simulink model "Crane3D"  (R2024b)
settings: Solver=ode4  StartTime=0.0  StopTime=Tsim  FixedStep=0.01  RelTol=1e-3  AbsTol=1e-6
values from neighbouring files (symbols this model uses):
  den_X = pCartd_X.den{1}    [script_3DCrane.m]
  den_Y = pCartd_Y.den{1}    [script_3DCrane.m]
  den_Z = pCartd_Z.den{1}    [script_3DCrane.m]
  num_X = pCartd_X.num{1}    [script_3DCrane.m]
  num_Y = pCartd_Y.num{1}    [script_3DCrane.m]
  num_Z = pCartd_Z.num{1}    [script_3DCrane.m]
  Ts = 0.01    [script_3DCrane.m]
libraries: simulink x1
settings Model: ExtModeTrigDuration=10000  Creator=jims  LastModifiedBy=David
settings SolverCC: AutoScaleAbsTol=off  AlgebraicLoopSolver=TrustRegion
settings DataIOCC: ExternalInput=[]  InitialState=[]  MaxDataPoints=5000  SaveFormat=Array  SaveOutput=off  SaveTime=off  ReturnWorkspaceOutputs=off
settings OptimizationCC: BooleanDataType=off  OptimizeBlockIOStorage=off  BufferReuse=off  GlobalBufferReuse=off  ExpressionFolding=off  ExpressionDepthLimit=2147483647  LocalBlockOutputs=off  InitFltsAndDblsToZero=on  LifeSpan=inf  OptimizeDataStoreBuffers=off  BusAssignmentInplaceUpdate=off
settings DebuggingCC: SaveWithParameterizedLinksMsg=none  UnderspecifiedInitializationDetection=Classic  MergeDetectMultiDrivingBlocksExec=none  SignalResolutionControl=TryResolveAllWithWarning  MultiTaskDSMMsg=warning  MultiTaskCondExecSysMsg=none  IntegerOverflowMsg=none  FcnCallInpInsideContextMsg=warning  UnconnectedInputMsg=warning  UnconnectedOutputMsg=warning  UnconnectedLineMsg=warning  StateNameClashWarn=warning  SFUnexpectedBacktrackingDiag=warning  SFNoUnconditionalDefaultTransitionDiag=warning  SFExecutionAtInitializationDiag=none  IntegerSaturationMsg=none  ArithmeticOperatorsInVariantConditions=warning
settings HardwareCC: ProdBitPerPointer=32  ProdBitPerSizeT=32  ProdBitPerPtrDiffT=32  ProdLargestAtomicFloat=None  ProdIntDivRoundTo=Undefined  ProdEndianess=Unspecified  ProdWordSize=32  ProdHWDeviceType=32-bit Generic
settings ModelReferenceCC: EnableRefExpFcnMdlSchedulingChecks=on  PropagateSignalLabelsOutOfModel=off
settings SFSimCC: SimUseLocalCustomCode=off  CustomCodeUndefinedFunction=UseInterfaceOnly
settings RTWCC: RTWUseLocalCustomCode=off  GPUComputeCapability=3.5
settings CodeAppCC: StateflowObjectComments=on
settings GRTTargetCC: TargetFcnLib=ansi_tfl_tmw.mat  TargetLangStandard=C89/C90 (ANSI)  CombineOutputUpdateFcns=off  GRTInterface=on
settings ConfigComp: CovMetricSettings=dw  CovSaveCumulativeToWorkspaceVar=on  CovSaveSingleToWorkspaceVar=on  CovExternalEMLEnable=off

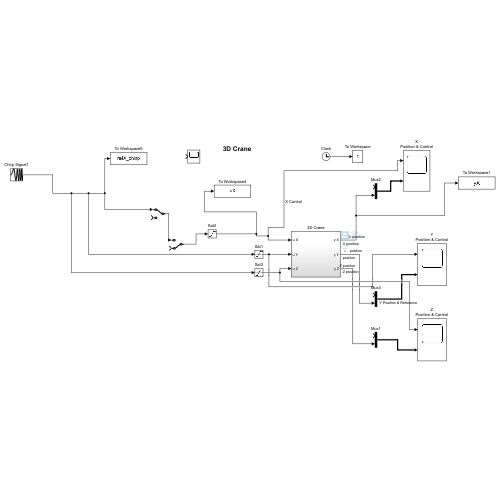
[thumbnail: Simulink's stored preview of the top-level diagram]
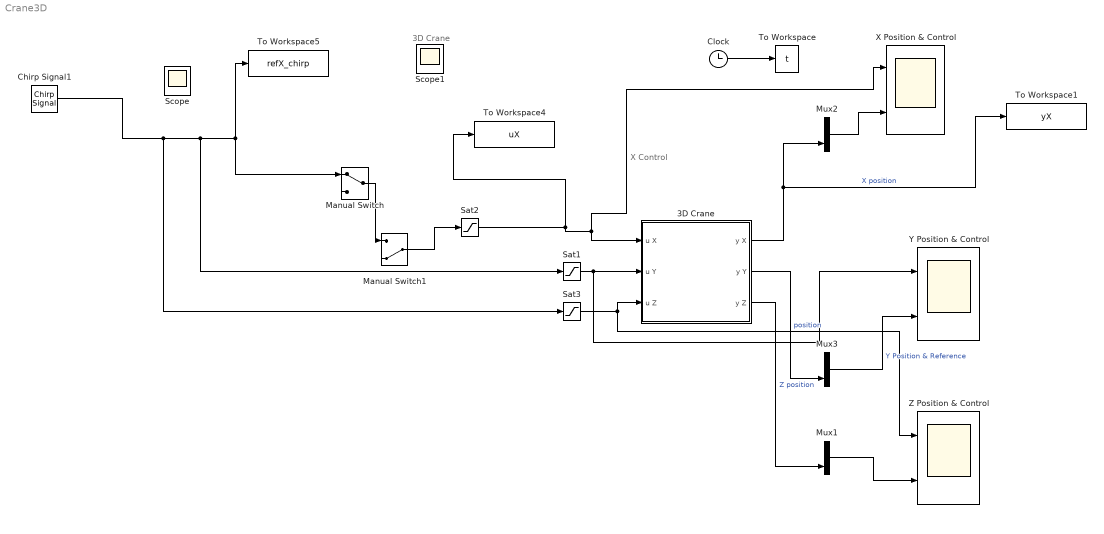
== system Crane3D ==
  note: 3D Crane
  note: X Control
  3D Crane : Subsystem
  Chirp Signal1 : simulink/Sources/Chirp Signal  f1=0.1  T=100  f2=1
  Clock : Clock
  Manual Switch : ManualSwitch
  Manual Switch1 : ManualSwitch  CurrentSetting=0
  Mux1 : Mux  Inputs=2
  Mux2 : Mux  Inputs=2
  Mux3 : Mux  Inputs=2
  Sat1 : Saturate  UpperLimit=1  LowerLimit=-1  SampleTime=Ts
  Sat2 : Saturate  UpperLimit=1  LowerLimit=-1  SampleTime=Ts
  Sat3 : Saturate  UpperLimit=1  LowerLimit=-1  SampleTime=Ts
  Scope1 : Scope
  To Workspace : ToWorkspace  VariableName=t  SampleTime=Ts
  To Workspace1 : ToWorkspace  VariableName=yX  SampleTime=Ts
      settings: Save2DSignal=2-D array (concatenate along first dimension)
  To Workspace4 : ToWorkspace  VariableName=uX  SampleTime=Ts
      settings: Save2DSignal=2-D array (concatenate along first dimension)
  To Workspace5 : ToWorkspace  VariableName=refX_chirp  SampleTime=Ts
      settings: Save2DSignal=2-D array (concatenate along first dimension)
  X Position & Control : Scope  NumInputPorts=2
  Y Position & Control : Scope  NumInputPorts=2
  Z Position & Control : Scope  NumInputPorts=2
  Scope : Scope
  wires:
  Mux2/1 -> X Position & Control/2
  Mux3/1 -> Y Position & Control/2  "Y Position & Reference"
  Clock/1 -> To Workspace/1
  Sat2/1 -> 3D Crane/1(u X), X Position & Control/1, To Workspace4/1
  Sat1/1 -> Y Position & Control/1, 3D Crane/2(u Y)
  Sat3/1 -> 3D Crane/3(u Z), Z Position & Control/1
  Mux1/1 -> Z Position & Control/2
  3D Crane/1(y X) -> To Workspace1/1, Mux2/2  "X position"
  3D Crane/2(y Y) -> Mux3/2  "position"
  3D Crane/3(y Z) -> Mux1/2  "Z position"
  Chirp Signal1/1 -> Sat3/1, Sat1/1, To Workspace5/1, Manual Switch/1
  Manual Switch/1 -> Manual Switch1/1
  Manual Switch1/1 -> Sat2/1

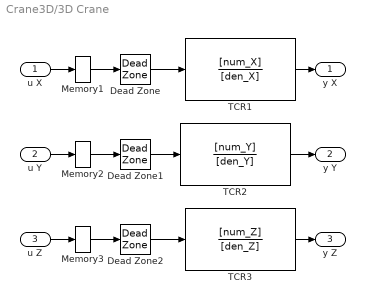
== system Crane3D/3D Crane ==
  u X : Inport
  u Y : Inport  Port=2
  u Z : Inport  Port=3
  Dead Zone : DeadZone  LowerValue=DZmin_X  UpperValue=DZmax_X
  Dead Zone1 : DeadZone  LowerValue=DZmin_Y  UpperValue=DZmax_Y
  Dead Zone2 : DeadZone  LowerValue=DZmin_Z  UpperValue=DZmax_Z
  Memory1 : Memory
  Memory2 : Memory
  Memory3 : Memory
  TCR1 : DiscreteTransferFcn  Numerator=[num_X]  Denominator=[den_X]  SampleTime=Ts
  TCR2 : DiscreteTransferFcn  Numerator=[num_Y]  Denominator=[den_Y]  SampleTime=Ts
  TCR3 : DiscreteTransferFcn  Numerator=[num_Z]  Denominator=[den_Z]  SampleTime=Ts
  y X : Outport  VectorParamsAs1DForOutWhenUnconnected=off
  y Y : Outport  Port=2  VectorParamsAs1DForOutWhenUnconnected=off
  y Z : Outport  Port=3  VectorParamsAs1DForOutWhenUnconnected=off
  wires:
  TCR2/1 -> y Y/1
  u Y/1 -> Memory2/1
  u X/1 -> Memory1/1
  TCR1/1 -> y X/1
  Dead Zone/1 -> TCR1/1
  Memory1/1 -> Dead Zone/1
  Dead Zone1/1 -> TCR2/1
  Memory2/1 -> Dead Zone1/1
  u Z/1 -> Memory3/1
  TCR3/1 -> y Z/1
  Dead Zone2/1 -> TCR3/1
  Memory3/1 -> Dead Zone2/1
